simulink model "block_ads"  (R2013a)
settings: Solver=ode45  StartTime=0.0  StopTime=2  RelTol=1e-3
undefined symbols (not defined in the file or in its folder): dfilt, fdesignblkfcn, gcbh
libraries: dsparch4 x3, visiontransforms x1, alsalib x1, dspsrcs4 x1, RCTblocks x1, simulink_extras x1, dspsnks4 x1
settings Model: Creator=mainster  LastModifiedBy=mainster

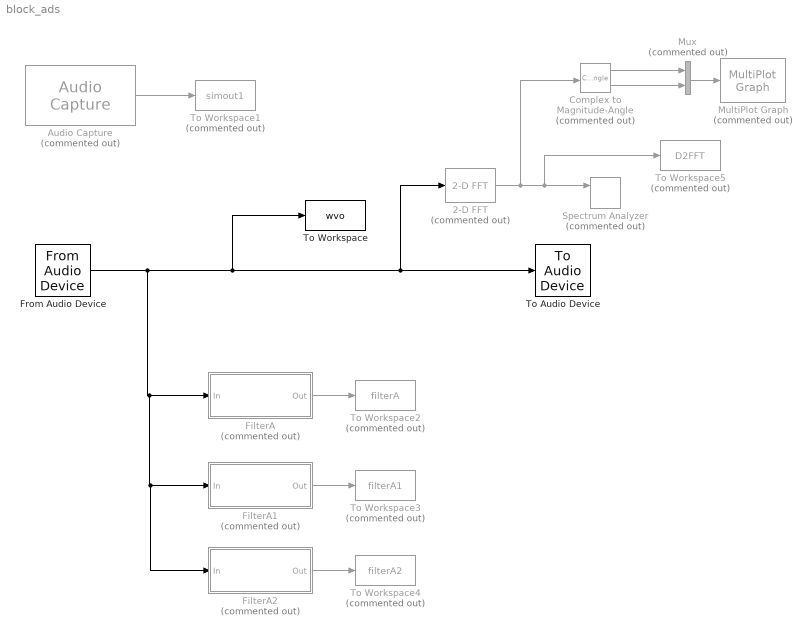
== system block_ads ==
  2-D FFT : visiontransforms/2-D FFT  Commented=on  TableOpt=NEW  TableOptActive=Speed  BitRevOrder=off  SkipNorm=on  FFTImplementation=Auto  firstCoeffDataTypeStr=Inherit: Same word length as input  firstCoeffLastDataTypeStr=Inherit: Same word length as input  outputMin=[]  outputMax=[]  roundingMode=Floor  overflowMode=off
  Audio Capture : alsalib/Audio Capture  Commented=on  deviceStr='default'  sampleRate=44100  queueDuration=0.5  frameSize=4096
  Complex to Magnitude-Angle : ComplexToMagnitudeAngle  Commented=on
  FilterA : Subsystem  Commented=on  DialogController=fdesignblkfcn  InitFcn=fdesignblkfcn(gcbh, {'InitFcn'});  mask(Audio Weighting Filter){}
      mask help: Design an audio weighting filter
      settings: CopyFcn=fdesignblkfcn(gcbh, {'CopyFcn'});
      mask Help: helpview(mapfilelocation('dsp'), 'dspaudioweightingfilter');
      mask Display: disp('Audio Weighting')
  FilterA1 : Subsystem  Commented=on  DialogController=fdesignblkfcn  InitFcn=fdesignblkfcn(gcbh, {'InitFcn'});  mask(Audio Weighting Filter){}
      mask help: Design an audio weighting filter
      settings: CopyFcn=fdesignblkfcn(gcbh, {'CopyFcn'});
      mask Help: helpview(mapfilelocation('dsp'), 'dspaudioweightingfilter');
      mask Display: disp('Audio Weighting')
  FilterA2 : Subsystem  Commented=on  DialogController=fdesignblkfcn  InitFcn=fdesignblkfcn(gcbh, {'InitFcn'});  mask(Audio Weighting Filter){}
      mask help: Design an audio weighting filter
      settings: CopyFcn=fdesignblkfcn(gcbh, {'CopyFcn'});
      mask Help: helpview(mapfilelocation('dsp'), 'dspaudioweightingfilter');
      mask Display: disp('Audio Weighting')
  From Audio Device : dspsrcs4/From Audio Device  RequirementInfo="{}  %GIDa_fa7561d9_893f_44b3_9f41_24b7397a2382"  deviceName=Default  numChannels=1  sampleRate=fs  deviceDatatype=16-bit integer  autoBufferSize=on  bufferSize=4096  queueDuration=1.0  frameSize=1024  outputDatatype=single
  MultiPlot Graph : RCTblocks/MultiPlot Graph  Tag=MultiPlot  Commented=on  tmin=0  tmax=1  ymin=-0.0036  ymax=0.0036  Tsamp=fs  vnamesave=multisimout
  Mux : Mux  Commented=on  Inputs=2
  Spectrum Analyzer : simulink_extras/Additional Sinks/Spectrum Analyzer  Commented=on  npts=256  fftpts=256  HowOften=64  sampleT=fs
  To Audio Device : dspsnks4/To Audio Device  deviceName=Default  inheritSampleRate=on  sampleRate=44100  deviceDatatype=Determine from input data type  autoBufferSize=on  bufferSize=4096  queueDuration=2
  To Workspace : ToWorkspace  VariableName=wvo  SampleTime=-1  SaveFormat=Timeseries
  To Workspace1 : ToWorkspace  Commented=on  VariableName=simout1  SampleTime=-1  SaveFormat=Timeseries
  To Workspace2 : ToWorkspace  Commented=on  VariableName=filterA  SampleTime=-1  SaveFormat=Timeseries
  To Workspace3 : ToWorkspace  Commented=on  VariableName=filterA1  SampleTime=-1  SaveFormat=Timeseries
  To Workspace4 : ToWorkspace  Commented=on  VariableName=filterA2  SampleTime=-1  SaveFormat=Timeseries
  To Workspace5 : ToWorkspace  Commented=on  VariableName=D2FFT  SampleTime=-1  SaveFormat=Timeseries
  wires:
  Audio Capture/1 -> To Workspace1/1
  FilterA/1(Out) -> To Workspace2/1
  FilterA1/1(Out) -> To Workspace3/1
  FilterA2/1(Out) -> To Workspace4/1
  From Audio Device/1 -> FilterA2/1(In), FilterA1/1(In), FilterA/1(In), To Workspace/1, 2-D FFT/1, To Audio Device/1
  Complex to Magnitude-Angle/1 -> Mux/1
  Complex to Magnitude-Angle/2 -> Mux/2
  Mux/1 -> MultiPlot Graph/1
  2-D FFT/1 -> Complex to Magnitude-Angle/1, To Workspace5/1, Spectrum Analyzer/1

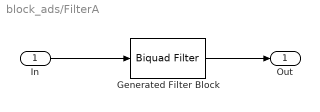
== system block_ads/FilterA ==
  In : Inport
  Generated Filter Block : dsparch4/Biquad Filter  Tag=BlockMethodSubSystem  IIRFiltStruct=Direct form II  CoeffSource=Specify via dialog  BiQuadCoeffs=[0.0150170119615565274 0.0300340239231130547 0.0150170119615565274 1 0.821563817981106448 0.168741776753923156;1 -2 1 1 -1.70550963370528952 0.715987575345399363;1 -2 1 1 -1.98388675726797903 0.98395166641581433]  a0Flag=Warning  IC=0  ICnum=0  ICden=0  InputProcessing=Columns as channels (frame based)  denAccumFracLength=30  denProdOutputFracLength=30  secondMemoryFracLength=15  roundingMode=Floor  overflowMode=off  ScaleValues=[0.347178019185922171;1;1;101.943422753540929]  optimizeScaleValues=off  ScaleValueMode=Specify via input port (g)  scaleValueFracLength=14  FilterSource=Specify via dialog  dfiltObjectName=dfilt.df2tsos([1 0.3 0.4],[1 0.1 0.2])
  Out : Outport
  wires:
  In/1 -> Generated Filter Block/1
  Generated Filter Block/1 -> Out/1

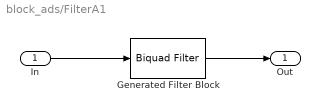
== system block_ads/FilterA1 ==
  In : Inport
  Generated Filter Block : dsparch4/Biquad Filter  Tag=BlockMethodSubSystem  IIRFiltStruct=Direct form II  CoeffSource=Specify via dialog  BiQuadCoeffs=[0.0150170119615565274 0.0300340239231130547 0.0150170119615565274 1 0.821563817981106448 0.168741776753923156;1 -2 1 1 -1.70550963370528952 0.715987575345399363;1 -2 1 1 -1.98388675726797903 0.98395166641581433]  a0Flag=Warning  IC=0  ICnum=0  ICden=0  InputProcessing=Columns as channels (frame based)  denAccumFracLength=30  denProdOutputFracLength=30  secondMemoryFracLength=15  roundingMode=Floor  overflowMode=off  ScaleValues=[0.347178019185922171;1;1;101.943422753540929]  optimizeScaleValues=off  ScaleValueMode=Specify via input port (g)  scaleValueFracLength=14  FilterSource=Specify via dialog  dfiltObjectName=dfilt.df2tsos([1 0.3 0.4],[1 0.1 0.2])
  Out : Outport
  wires:
  In/1 -> Generated Filter Block/1
  Generated Filter Block/1 -> Out/1

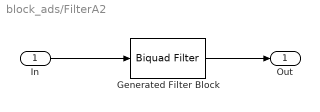
== system block_ads/FilterA2 ==
  In : Inport
  Generated Filter Block : dsparch4/Biquad Filter  Tag=BlockMethodSubSystem  IIRFiltStruct=Direct form II  CoeffSource=Specify via dialog  BiQuadCoeffs=[0.0150170119615565274 0.0300340239231130547 0.0150170119615565274 1 0.821563817981106448 0.168741776753923156;1 -2 1 1 -1.70550963370528952 0.715987575345399363;1 -2 1 1 -1.98388675726797903 0.98395166641581433]  a0Flag=Warning  IC=0  ICnum=0  ICden=0  InputProcessing=Columns as channels (frame based)  denAccumFracLength=30  denProdOutputFracLength=30  secondMemoryFracLength=15  roundingMode=Floor  overflowMode=off  ScaleValues=[0.347178019185922171;1;1;101.943422753540929]  optimizeScaleValues=off  ScaleValueMode=Specify via input port (g)  scaleValueFracLength=14  FilterSource=Specify via dialog  dfiltObjectName=dfilt.df2tsos([1 0.3 0.4],[1 0.1 0.2])
  Out : Outport
  wires:
  In/1 -> Generated Filter Block/1
  Generated Filter Block/1 -> Out/1
